simulink model "prova"  (R2017b)
settings: Solver=FixedStepDiscrete  StartTime=0.0  StopTime=10.0  FixedStep=0.1  RelTol=1e-3  EnableMultiTasking=on
settings Model: Creator=Fabio  LastModifiedBy=Fabio
settings SolverCC: AutoInsertRateTranBlk=on
settings DataIOCC: LimitDataPoints=on
settings OptimizationCC: LifeSpan=inf
settings DebuggingCC: AllowSymbolicDim=off  SFUnexpectedBacktrackingDiag=warning  SFNoUnconditionalDefaultTransitionDiag=warning  SFExecutionAtInitializationDiag=none
settings CodeAppCC: StateflowObjectComments=on
settings GRTTargetCC: TargetLangStandard=C89/C90 (ANSI)
settings ConfigComp: CovMetricSettings=dw  CovHtmlReporting=on  CovSaveCumulativeToWorkspaceVar=on  CovSaveSingleToWorkspaceVar=on  CovShowResultsExplorer=off  CovExternalEMLEnable=off

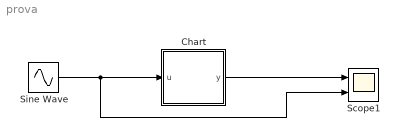
== system prova ==
  Chart : Stateflow chart  TreatAsAtomicUnit=on
  Scope1 : Scope  NumInputPorts=2
  Sine Wave : Sin  SampleTime=0
  wires:
  Sine Wave/1 -> Scope1/2, Chart/1(u)
  Chart/1(y) -> Scope1/1

== stateflow chart prova/Chart ==
  state State2
    during: y=decrement(y)
  state State1 %State Name
    entry: y = 0; % entry action
    during: y=increment(y);
  (default) -> State1 %State Name
  State1 %State Name -> State2 : [u <= 0]
      | % [transition condition]{action}
  State2 -> State1 %State Name : [u > 0]
  data: val function_input; sum function_output; val function_input; dec function_output; u input; y output
  function sum=increment(val):
    | function sum=increment(val)
    | 
    | sum=val+1;
  function dec=decrement(val):
    | function dec=decrement(val)
    | dec=val-1;
